simulink model "amalifuzzypidzoptimal"  (R2021a)
settings: Solver=FixedStepAuto  StartTime=0.0  StopTime=60  RelTol=1e-2
InitFcn:
  | Ts=0.01;
  | 
  | Kpmin1 = 3;
  | Kpmax1 = 12;
  | Kdmin1 = 3;
  | Kdmax1 = 11;
  | 
  | Kpmin2 = 3;
  | Kpmax2 = 11;
  | Kdmin2 = 3;
  | Kdmax2 = 10;
  | 
  | Kpmin = 3;
  | Kpmax = 13;
  | Kdmin = 4;
  | Kdmax = 12;
libraries: raspberrypiCommlib x6, pid_lib x4, raspberrypiBasiclib x4, fuzblock x3, simulink_extras x2, etargetslib x1, raspberrypiNetworklib x1
settings Model: Creator=pouria  LastModifiedBy=pouria
settings SolverCC: AlgebraicLoopSolver=TrustRegion  PositivePriorityOrder=on  AutoInsertRateTranBlk=on
settings DataIOCC: LimitDataPoints=on  SaveFormat=Array  ReturnWorkspaceOutputs=off
settings OptimizationCC: EnhancedBackFolding=on  PassReuseOutputArgsAs=Individual arguments  ZeroExternalMemoryAtStartup=off  ZeroInternalMemoryAtStartup=off  MaxStackSize=64  OptimizeBlockOrder=speed  DifferentSizesBufferReuse=on  OptimizationCustomize=off  EfficientTunableParamExpr=on
settings DebuggingCC: ParameterTunabilityLossMsg=error  SFUnexpectedBacktrackingDiag=warning  SFNoUnconditionalDefaultTransitionDiag=warning  SFExecutionAtInitializationDiag=none  SFMachineParentedDataDiag=warning  ArithmeticOperatorsInVariantConditions=warning
settings HardwareCC: ProdBitPerPointer=32  ProdBitPerSizeT=32  ProdBitPerPtrDiffT=32  ProdLargestAtomicInteger=Long  ProdLargestAtomicFloat=Double  ProdWordSize=32  ProdLongLongMode=on  ProdHWDeviceType=ARM Compatible->ARM Cortex
settings ModelReferenceCC: PropagateSignalLabelsOutOfModel=off
settings SFSimCC: SimUseLocalCustomCode=off  CustomCodeUndefinedFunction=UseInterfaceOnly
settings RTWCC: SystemTargetFile=ert.tlc  HardwareBoard=Raspberry Pi  TLCOptions="-aInlineSetEventsForThisBaseRateFcn=TLC_FALSE -aSuppressMultiTaskScheduler=TLC_FALSE  -aRateBasedStepFcn=0"  TemplateMakefile=ert_default_tmf  RTWUseLocalCustomCode=off  Toolchain=GNU GCC Embedded Linux  BuildConfiguration=Faster Runs
settings CodeAppCC: ForceParamTrailComments=on  IgnoreCustomStorageClasses=off  OperatorAnnotations=on  SimulinkDataObjDesc=on  SFDataObjDesc=on  InsertBlockDesc=on
settings ERTTargetCC: SupportContinuousTime=on  SupportVariableSizeSignals=on  ExtModeTransport=2  ExtModeStaticAlloc=on  ExtModeMexFile=ext_xcp  ExtModeIntrfLevel=Level2 - Open
settings ConfigComp: CovMetricSettings=dw  CovSaveCumulativeToWorkspaceVar=on  CovSaveSingleToWorkspaceVar=on  CovExternalEMLEnable=off  CovSFcnEnable=off

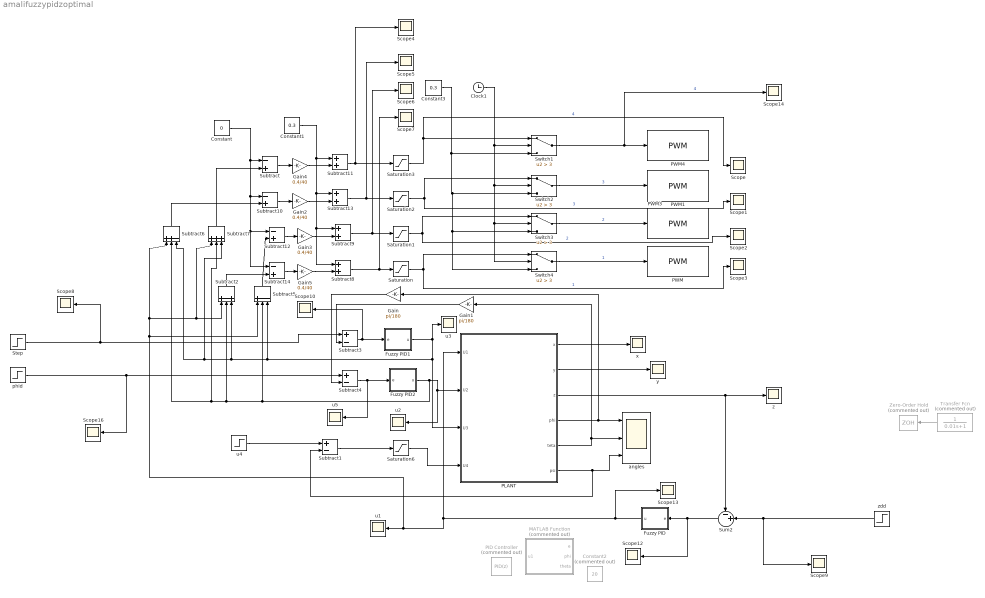
== system amalifuzzypidzoptimal ==
  Clock1 : Clock
  Constant : Constant  Value=0  SampleTime=Ts
  Constant1 : Constant  Value=0.3  SampleTime=Ts
  Constant2 : Constant  Commented=on  Value=20
  Constant3 : Constant  Value=0.3  SampleTime=Ts
  Fuzzy PID : Subsystem
  Fuzzy PID1 : Subsystem
  Fuzzy PID2 : Subsystem
  Gain : Gain  Gain=pi/180
  Gain1 : Gain  Gain=pi/180
  Gain{2..5} (4 alike) : Gain  Gain=0.4/40
  MATLAB Function : MATLAB Function  Commented=on  TreatAsAtomicUnit=on
  PID Controller : pid_lib/PID Controller  Commented=on  Controller=PID  Form=Parallel  TimeDomain=Discrete-time  UseExternalTs=off  SampleTime=0.01  IntegratorMethod=Backward Euler  FilterMethod=Backward Euler  ControllerParametersSource=internal  P=5  I=3  D=5  UseFilter=on  N=100  TunerSelectOption=Transfer Function Based (PID Tuner App)  InitialConditionSource=internal  InitialConditionForIntegrator=0  InitialConditionForFilter=0  DifferentiatorICPrevScaledInput=0  ExternalReset=none  TrackingMode=off  Kt=1  LimitOutput=off  SatLimitsSource=internal  UpperSaturationLimit=inf  LowerSaturationLimit=-inf  LinearizeAsGain=on  AntiWindupMode=none  Kb=1  POutMin=[]  POutMax=[]  IOutMin=[]  IOutMax=[]  DOutMin=[]  DOutMax=[]  NOutMin=[]  NOutMax=[]  SumOutMin=[]  SumOutMax=[]  SaturationOutMin=[]  SaturationOutMax=[]  PParamMin=[]  PParamMax=[]  IParamMin=[]  IParamMax=[]  DParamMin=[]  DParamMax=[]  NParamMin=[]  NParamMax=[]  KbParamMin=[]  KbParamMax=[]  KtParamMin=[]  KtParamMax=[]  KbOutMin=[]  KbOutMax=[]  KtOutMin=[]  KtOutMax=[]  IntegratorOutMin=[]  IntegratorOutMax=[]  FilterOutMin=[]  FilterOutMax=[]  SumI1OutMin=[]  SumI1OutMax=[]  SumI2OutMin=[]  SumI2OutMax=[]  SumI3OutMin=[]  SumI3OutMax=[]  SumI4OutMin=[]  SumI4OutMax=[]  SumDOutMin=[]  SumDOutMax=[]  DifferentiatorOutMin=[]  DifferentiatorOutMax=[]  FilterDiffOutCoefMin=[]  FilterDiffOutCoefMax=[]  ReciprocalOutMin=[]  ReciprocalOutMax=[]  SumDenOutMin=[]  SumDenOutMax=[]  SumNumOutMin=[]  SumNumOutMax=[]  DivideOutMin=[]  DivideOutMax=[]  UdiffTsProdOutMin=[]  UdiffTsProdOutMax=[]  NTsProdOutMin=[]  NTsProdOutMax=[]  UintegralTsProdOutMin=[]  UintegralTsProdOutMax=[]  UngainTsProdOutMin=[]  UngainTsProdOutMax=[]  IntegratorContinuousStateAttributes=''  IntegratorStateMustResolveToSignalObject=off  IntegratorRTWStateStorageClass=Auto  FilterContinuousStateAttributes=''  FilterStateMustResolveToSignalObject=off  FilterRTWStateStorageClass=Auto  ParallelPVariant=InternalParameters  IdealPVariant=Disabled  IVariant=InternalParameters  DVariant=InternalParameters  IntegratorVariant=Discrete  SatVariant=Disabled  AWVariant=Passthrough  PCopyVariant=Disabled  TRVariant=Disabled  FdbkBlocksVariant=Forward  IdealPFdbkVariant=Disabled  SatFdbkVariant=Disabled  DerivativeFilterVariant=BackwardEulerFilter  NVariant=InternalParameters  NCopyVariant=InternalParameters  FilterICVariant=InternalICsFilter  IntegratorICVariant=InternalICs  ExternalResetVariant=Disabled  TRSumVariant=Passthrough  SumFdbkVariant=Disabled  SumVariant=Sum_PID  TsampFilterVariant=InternalTs  TsampNgainVariant=Passthrough  TsampIntegralVariant=Passthrough  ExternalSaturationOutDataTypeStr=Inherit: Same as second input
  PLANT : Subsystem
  PWM : raspberrypiBasiclib/PWM  board=Pi 3 Model B  Pin_=21  Frequency=400  blockPlatform=Raspberry Pi
      settings: SourceProductBaseCode=RASPPI
  PWM1 : raspberrypiBasiclib/PWM  board=Pi 3 Model B  Pin_=20  Frequency=400  blockPlatform=Raspberry Pi
      settings: SourceProductBaseCode=RASPPI
  PWM3 : raspberrypiBasiclib/PWM  board=Pi 3 Model B  Pin_=16  Frequency=400  blockPlatform=Raspberry Pi
      settings: SourceProductBaseCode=RASPPI
  PWM4 : raspberrypiBasiclib/PWM  board=Pi 3 Model B  Pin_=19  Frequency=400  blockPlatform=Raspberry Pi
      settings: SourceProductBaseCode=RASPPI
  Saturation{,1..3} (4 alike) : Saturate  UpperLimit=0.7  LowerLimit=0.3
  Saturation6 : Saturate  UpperLimit=0  LowerLimit=0
  Scope{,1..10,12..14,16} (15 alike) : Scope
  Step : Step  Time=0  After=0  SampleTime=Ts
  Subtract{,10,12,14} (4 alike) : Sum  Inputs=-+
  Subtract1 : Sum  Inputs=+-
  Subtract{8..9,11,13} (4 alike) : Sum
  Subtract2 : Sum  Inputs=+-+
  Subtract3 : Sum  Inputs=+-
  Subtract4 : Sum  Inputs=+-
  Subtract5 : Sum  Inputs=+--
  Subtract6 : Sum  Inputs=++-
  Subtract7 : Sum  Inputs=+++
  Sum2 : Sum  Inputs=-+|
  Switch{1..4} (4 alike) : Switch  Criteria=u2 > Threshold  Threshold=3
  Transfer Fcn : TransferFcn  Commented=on  Denominator=[0.01 1]
  Zero-Order Hold : ZeroOrderHold  Commented=on  SampleTime=Ts
  angles : Scope  NumInputPorts=3
  phid : Step  Time=0  After=0  SampleTime=Ts
  u{1..3,5} (4 alike) : Scope
  u4 : Step  Time=0  After=0  SampleTime=Ts
  x : Scope
  y : Scope
  z : Scope
  zdd : Step  Time=5  Before=0.06  After=0.25  SampleTime=Ts
  wires:
  PLANT/6(psi) -> angles/3, Subtract1/2
  PLANT/1(x) -> x/1
  PLANT/2(y) -> y/1
  Subtract4/1 -> Fuzzy PID2/1(e), u5/1
  Subtract3/1 -> Fuzzy PID1/1(e), Scope10/1
  u4/1 -> Subtract1/1
  Subtract1/1 -> Saturation6/1
  PLANT/3(z) -> z/1, Sum2/1
  PLANT/4(phi) -> angles/1, Gain/1
  PLANT/5(teta) -> angles/2, Gain1/1
  Saturation/1 -> Switch4/1, Scope3/1  "1"
  Saturation1/1 -> Switch3/1, Scope2/1  "2"
  Saturation2/1 -> Switch2/1, Scope1/1  "3"
  Saturation3/1 -> Switch1/1, Scope/1  "4"
  Gain/1 -> Subtract4/2
  Gain1/1 -> Subtract3/2
  Saturation6/1 -> PLANT/4(U4)
  Subtract7/1 -> Subtract/2
  Subtract6/1 -> Subtract10/2
  Subtract5/1 -> Subtract12/2
  Constant/1 -> Subtract14/1, Subtract12/1, Subtract10/1, Subtract/1
  Subtract2/1 -> Subtract14/2
  Clock1/1 -> Switch4/2, Switch3/2, Switch2/2, Switch1/2
  Switch1/1 -> Scope14/1, PWM4/1  "4"
  Constant3/1 -> Switch1/3, Switch3/3, Switch4/3, Switch2/3
  Switch2/1 -> PWM1/1  "3"
  Switch3/1 -> PWM3/1  "2"
  Switch4/1 -> PWM/1  "1"
  Subtract9/1 -> Scope6/1, Saturation1/1
  Subtract13/1 -> Scope5/1, Saturation2/1
  Subtract11/1 -> Scope4/1, Saturation3/1
  Subtract8/1 -> Scope7/1, Saturation/1
  Subtract14/1 -> Gain5/1
  Subtract12/1 -> Gain3/1
  Subtract10/1 -> Gain2/1
  Subtract/1 -> Gain4/1
  Constant1/1 -> Subtract8/1, Subtract9/1, Subtract13/1, Subtract11/1
  Gain4/1 -> Subtract11/2
  Gain2/1 -> Subtract13/2
  Gain3/1 -> Subtract9/2
  Gain5/1 -> Subtract8/2
  Step/1 -> Scope8/1, Subtract3/1
  phid/1 -> Scope16/1, Subtract4/1
  Sum2/1 -> Fuzzy PID/1(e), Scope12/1
  Fuzzy PID1/1(u) -> PLANT/3(U3), Subtract5/3, Subtract2/3, Subtract6/3, Subtract7/3, u3/1
  Fuzzy PID2/1(u) -> u2/1, PLANT/2(U2), Subtract5/2, Subtract2/2, Subtract7/2, Subtract6/2
  Fuzzy PID/1(u) -> Scope13/1, Subtract5/1, Subtract2/1, Subtract7/1, Subtract6/1, u1/1, PLANT/1(U1)
  zdd/1 -> Scope9/1, Sum2/2
  Transfer Fcn/1 -> Zero-Order Hold/1

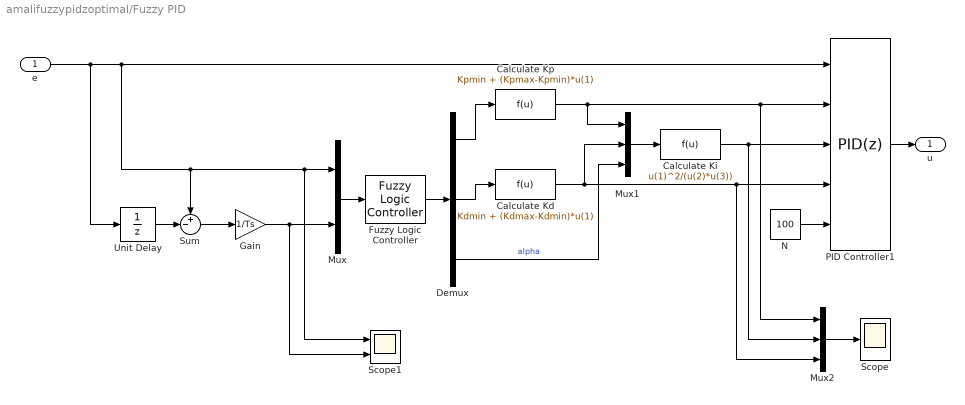
== system amalifuzzypidzoptimal/Fuzzy PID ==
  e : Inport
  Calculate Kd : Fcn  Expr=Kdmin + (Kdmax-Kdmin)*u(1)
  Calculate Ki : Fcn  Expr=u(1)^2/(u(2)*u(3))
  Calculate Kp : Fcn  Expr=Kpmin + (Kpmax-Kpmin)*u(1)
  Demux : Demux  Outputs=3
  Fuzzy Logic Controller : fuzblock/Fuzzy Logic  Controller  FIS='fuzzy_pid1.fis'  OutputSampleNumber=101  DataType=double  FuzzifiedInputs=off  RuleFiringStrengths=off  RuleOutputs=off  AggregatedOutputs=off  SimulateUsing=Interpreted execution  OutOfRangeInputValueMessage=warning  NoRuleFiredMessage=warning  EmptyOutputFuzzySetMessage=warning
  Gain : Gain  Gain=1/Ts
  Mux : Mux  Inputs=2
  Mux1 : Mux  Inputs=3
  Mux2 : Mux  Inputs=3
  N : Constant  Value=100
  PID Controller1 : pid_lib/PID Controller  Controller=PID  Form=Parallel  TimeDomain=Discrete-time  UseExternalTs=off  SampleTime=Ts  IntegratorMethod=Backward Euler  FilterMethod=Backward Euler  ControllerParametersSource=external  P=0.6*4.6737  I=1.2*4.6737/3.26  D=0.6*4.6737*3.26/8  UseFilter=on  N=100  TunerSelectOption=Transfer Function Based (PID Tuner App)  InitialConditionSource=internal  InitialConditionForIntegrator=0  InitialConditionForFilter=0  DifferentiatorICPrevScaledInput=0  ExternalReset=none  TrackingMode=off  Kt=1  LimitOutput=off  SatLimitsSource=internal  UpperSaturationLimit=inf  LowerSaturationLimit=-inf  LinearizeAsGain=on  AntiWindupMode=none  Kb=1  POutMin=[]  POutMax=[]  IOutMin=[]  IOutMax=[]  DOutMin=[]  DOutMax=[]  NOutMin=[]  NOutMax=[]  SumOutMin=[]  SumOutMax=[]  SaturationOutMin=[]  SaturationOutMax=[]  PParamMin=[]  PParamMax=[]  IParamMin=[]  IParamMax=[]  DParamMin=[]  DParamMax=[]  NParamMin=[]  NParamMax=[]  KbParamMin=[]  KbParamMax=[]  KtParamMin=[]  KtParamMax=[]  KbOutMin=[]  KbOutMax=[]  KtOutMin=[]  KtOutMax=[]  IntegratorOutMin=[]  IntegratorOutMax=[]  FilterOutMin=[]  FilterOutMax=[]  SumI1OutMin=[]  SumI1OutMax=[]  SumI2OutMin=[]  SumI2OutMax=[]  SumI3OutMin=[]  SumI3OutMax=[]  SumI4OutMin=[]  SumI4OutMax=[]  SumDOutMin=[]  SumDOutMax=[]  DifferentiatorOutMin=[]  DifferentiatorOutMax=[]  FilterDiffOutCoefMin=[]  FilterDiffOutCoefMax=[]  ReciprocalOutMin=[]  ReciprocalOutMax=[]  SumDenOutMin=[]  SumDenOutMax=[]  SumNumOutMin=[]  SumNumOutMax=[]  DivideOutMin=[]  DivideOutMax=[]  UdiffTsProdOutMin=[]  UdiffTsProdOutMax=[]  NTsProdOutMin=[]  NTsProdOutMax=[]  UintegralTsProdOutMin=[]  UintegralTsProdOutMax=[]  UngainTsProdOutMin=[]  UngainTsProdOutMax=[]  IntegratorContinuousStateAttributes=''  IntegratorStateMustResolveToSignalObject=off  IntegratorRTWStateStorageClass=Auto  FilterContinuousStateAttributes=''  FilterStateMustResolveToSignalObject=off  FilterRTWStateStorageClass=Auto  ParallelPVariant=ExternalParameters  IdealPVariant=Disabled  IVariant=ExternalParameters  DVariant=ExternalParameters  IntegratorVariant=Discrete  SatVariant=Disabled  AWVariant=Passthrough  PCopyVariant=Disabled  TRVariant=Disabled  FdbkBlocksVariant=Forward  IdealPFdbkVariant=Disabled  SatFdbkVariant=Disabled  DerivativeFilterVariant=BackwardEulerFilter  NVariant=ExternalParameters  NCopyVariant=ExternalParameters  FilterICVariant=InternalICsFilter  IntegratorICVariant=InternalICs  ExternalResetVariant=Disabled  TRSumVariant=Passthrough  SumFdbkVariant=Disabled  SumVariant=Sum_PID  TsampFilterVariant=InternalTs  TsampNgainVariant=Passthrough  TsampIntegralVariant=Passthrough  ExternalSaturationOutDataTypeStr=Inherit: Same as second input
  Scope : Scope
  Scope1 : Scope  NumInputPorts=2
  Sum : Sum  Inputs=+-|
  Unit Delay : UnitDelay  SampleTime=Ts  HasFrameUpgradeWarning=on
  u : Outport
  wires:
  PID Controller1/1 -> u/1
  N/1 -> PID Controller1/5
  Mux/1 -> Fuzzy Logic Controller/1
  Fuzzy Logic Controller/1 -> Demux/1
  Demux/1 -> Calculate Kp/1
  Calculate Kp/1 -> Mux2/1, PID Controller1/2, Mux1/1
  Demux/2 -> Calculate Kd/1
  Calculate Kd/1 -> Mux1/2, Mux2/3, PID Controller1/4
  Calculate Ki/1 -> Mux2/2, PID Controller1/3
  Mux1/1 -> Calculate Ki/1
  Demux/3 -> Mux1/3  "alpha"
  Unit Delay/1 -> Sum/2
  Mux2/1 -> Scope/1
  e/1 -> Unit Delay/1, Sum/1, Scope1/1, Mux/1, PID Controller1/1
  Sum/1 -> Gain/1
  Gain/1 -> Scope1/2, Mux/2

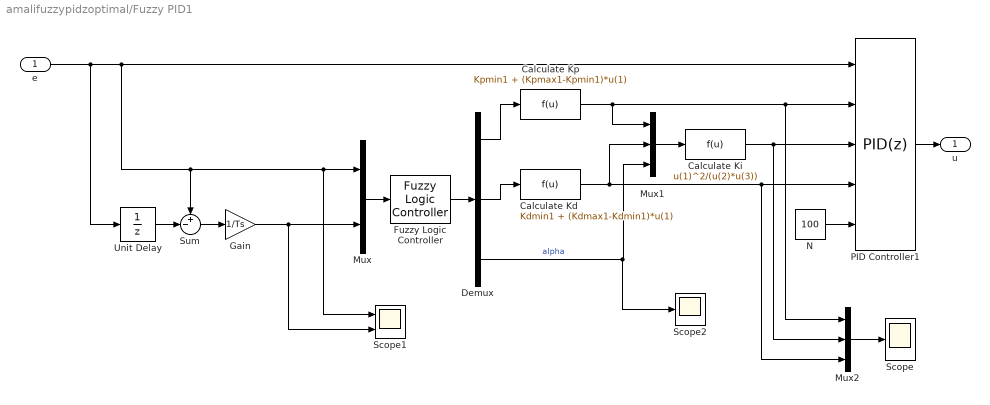
== system amalifuzzypidzoptimal/Fuzzy PID1 ==
  e : Inport
  Calculate Kd : Fcn  Expr=Kdmin1 + (Kdmax1-Kdmin1)*u(1)
  Calculate Ki : Fcn  Expr=u(1)^2/(u(2)*u(3))
  Calculate Kp : Fcn  Expr=Kpmin1 + (Kpmax1-Kpmin1)*u(1)
  Demux : Demux  Outputs=3
  Fuzzy Logic Controller : fuzblock/Fuzzy Logic  Controller  FIS='fuzzy_pidzavie.fis'  OutputSampleNumber=101  DataType=double  FuzzifiedInputs=off  RuleFiringStrengths=off  RuleOutputs=off  AggregatedOutputs=off  SimulateUsing=Interpreted execution  OutOfRangeInputValueMessage=warning  NoRuleFiredMessage=warning  EmptyOutputFuzzySetMessage=warning
  Gain : Gain  Gain=1/Ts
  Mux : Mux  Inputs=2
  Mux1 : Mux  Inputs=3
  Mux2 : Mux  Inputs=3
  N : Constant  Value=100
  PID Controller1 : pid_lib/PID Controller  Controller=PID  Form=Parallel  TimeDomain=Discrete-time  UseExternalTs=off  SampleTime=Ts  IntegratorMethod=Backward Euler  FilterMethod=Backward Euler  ControllerParametersSource=external  P=0.6*4.6737  I=1.2*4.6737/3.26  D=0.6*4.6737*3.26/8  UseFilter=on  N=100  TunerSelectOption=Transfer Function Based (PID Tuner App)  InitialConditionSource=internal  InitialConditionForIntegrator=0  InitialConditionForFilter=0  DifferentiatorICPrevScaledInput=0  ExternalReset=none  TrackingMode=off  Kt=1  LimitOutput=off  SatLimitsSource=internal  UpperSaturationLimit=inf  LowerSaturationLimit=-inf  LinearizeAsGain=on  AntiWindupMode=none  Kb=1  POutMin=[]  POutMax=[]  IOutMin=[]  IOutMax=[]  DOutMin=[]  DOutMax=[]  NOutMin=[]  NOutMax=[]  SumOutMin=[]  SumOutMax=[]  SaturationOutMin=[]  SaturationOutMax=[]  PParamMin=[]  PParamMax=[]  IParamMin=[]  IParamMax=[]  DParamMin=[]  DParamMax=[]  NParamMin=[]  NParamMax=[]  KbParamMin=[]  KbParamMax=[]  KtParamMin=[]  KtParamMax=[]  KbOutMin=[]  KbOutMax=[]  KtOutMin=[]  KtOutMax=[]  IntegratorOutMin=[]  IntegratorOutMax=[]  FilterOutMin=[]  FilterOutMax=[]  SumI1OutMin=[]  SumI1OutMax=[]  SumI2OutMin=[]  SumI2OutMax=[]  SumI3OutMin=[]  SumI3OutMax=[]  SumI4OutMin=[]  SumI4OutMax=[]  SumDOutMin=[]  SumDOutMax=[]  DifferentiatorOutMin=[]  DifferentiatorOutMax=[]  FilterDiffOutCoefMin=[]  FilterDiffOutCoefMax=[]  ReciprocalOutMin=[]  ReciprocalOutMax=[]  SumDenOutMin=[]  SumDenOutMax=[]  SumNumOutMin=[]  SumNumOutMax=[]  DivideOutMin=[]  DivideOutMax=[]  UdiffTsProdOutMin=[]  UdiffTsProdOutMax=[]  NTsProdOutMin=[]  NTsProdOutMax=[]  UintegralTsProdOutMin=[]  UintegralTsProdOutMax=[]  UngainTsProdOutMin=[]  UngainTsProdOutMax=[]  IntegratorContinuousStateAttributes=''  IntegratorStateMustResolveToSignalObject=off  IntegratorRTWStateStorageClass=Auto  FilterContinuousStateAttributes=''  FilterStateMustResolveToSignalObject=off  FilterRTWStateStorageClass=Auto  ParallelPVariant=ExternalParameters  IdealPVariant=Disabled  IVariant=ExternalParameters  DVariant=ExternalParameters  IntegratorVariant=Discrete  SatVariant=Disabled  AWVariant=Passthrough  PCopyVariant=Disabled  TRVariant=Disabled  FdbkBlocksVariant=Forward  IdealPFdbkVariant=Disabled  SatFdbkVariant=Disabled  DerivativeFilterVariant=BackwardEulerFilter  NVariant=ExternalParameters  NCopyVariant=ExternalParameters  FilterICVariant=InternalICsFilter  IntegratorICVariant=InternalICs  ExternalResetVariant=Disabled  TRSumVariant=Passthrough  SumFdbkVariant=Disabled  SumVariant=Sum_PID  TsampFilterVariant=InternalTs  TsampNgainVariant=Passthrough  TsampIntegralVariant=Passthrough  ExternalSaturationOutDataTypeStr=Inherit: Same as second input
  Scope : Scope
  Scope1 : Scope  NumInputPorts=2
  Scope2 : Scope
  Sum : Sum  Inputs=+-|
  Unit Delay : UnitDelay  SampleTime=Ts  HasFrameUpgradeWarning=on
  u : Outport
  wires:
  PID Controller1/1 -> u/1
  N/1 -> PID Controller1/5
  Mux/1 -> Fuzzy Logic Controller/1
  Fuzzy Logic Controller/1 -> Demux/1
  Demux/1 -> Calculate Kp/1
  Calculate Kp/1 -> Mux2/1, PID Controller1/2, Mux1/1
  Demux/2 -> Calculate Kd/1
  Calculate Kd/1 -> Mux1/2, Mux2/3, PID Controller1/4
  Calculate Ki/1 -> Mux2/2, PID Controller1/3
  Mux1/1 -> Calculate Ki/1
  Demux/3 -> Scope2/1, Mux1/3  "alpha"
  Unit Delay/1 -> Sum/2
  Mux2/1 -> Scope/1
  e/1 -> Unit Delay/1, Sum/1, Scope1/1, Mux/1, PID Controller1/1
  Sum/1 -> Gain/1
  Gain/1 -> Scope1/2, Mux/2

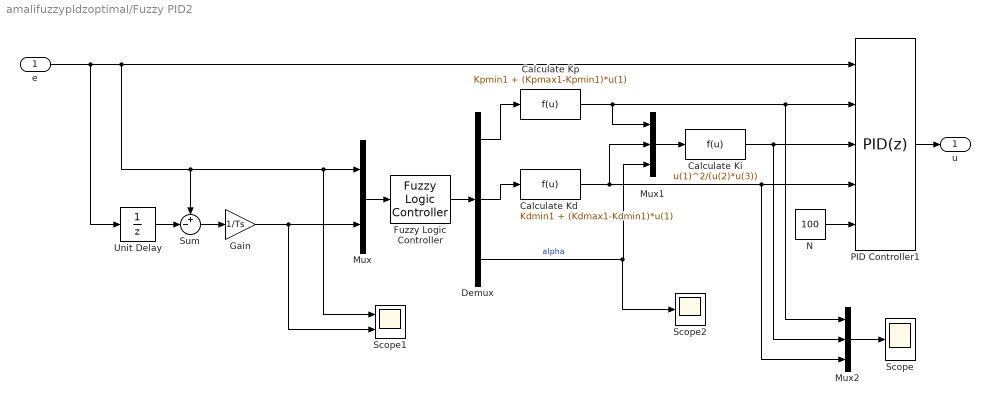
== system amalifuzzypidzoptimal/Fuzzy PID2 ==
  e : Inport
  Calculate Kd : Fcn  Expr=Kdmin1 + (Kdmax1-Kdmin1)*u(1)
  Calculate Ki : Fcn  Expr=u(1)^2/(u(2)*u(3))
  Calculate Kp : Fcn  Expr=Kpmin1 + (Kpmax1-Kpmin1)*u(1)
  Demux : Demux  Outputs=3
  Fuzzy Logic Controller : fuzblock/Fuzzy Logic  Controller  FIS='fuzzy_pidzavie.fis'  OutputSampleNumber=101  DataType=double  FuzzifiedInputs=off  RuleFiringStrengths=off  RuleOutputs=off  AggregatedOutputs=off  SimulateUsing=Interpreted execution  OutOfRangeInputValueMessage=warning  NoRuleFiredMessage=warning  EmptyOutputFuzzySetMessage=warning
  Gain : Gain  Gain=1/Ts
  Mux : Mux  Inputs=2
  Mux1 : Mux  Inputs=3
  Mux2 : Mux  Inputs=3
  N : Constant  Value=100
  PID Controller1 : pid_lib/PID Controller  Controller=PID  Form=Parallel  TimeDomain=Discrete-time  UseExternalTs=off  SampleTime=Ts  IntegratorMethod=Backward Euler  FilterMethod=Backward Euler  ControllerParametersSource=external  P=0.6*4.6737  I=1.2*4.6737/3.26  D=0.6*4.6737*3.26/8  UseFilter=on  N=100  TunerSelectOption=Transfer Function Based (PID Tuner App)  InitialConditionSource=internal  InitialConditionForIntegrator=0  InitialConditionForFilter=0  DifferentiatorICPrevScaledInput=0  ExternalReset=none  TrackingMode=off  Kt=1  LimitOutput=off  SatLimitsSource=internal  UpperSaturationLimit=inf  LowerSaturationLimit=-inf  LinearizeAsGain=on  AntiWindupMode=none  Kb=1  POutMin=[]  POutMax=[]  IOutMin=[]  IOutMax=[]  DOutMin=[]  DOutMax=[]  NOutMin=[]  NOutMax=[]  SumOutMin=[]  SumOutMax=[]  SaturationOutMin=[]  SaturationOutMax=[]  PParamMin=[]  PParamMax=[]  IParamMin=[]  IParamMax=[]  DParamMin=[]  DParamMax=[]  NParamMin=[]  NParamMax=[]  KbParamMin=[]  KbParamMax=[]  KtParamMin=[]  KtParamMax=[]  KbOutMin=[]  KbOutMax=[]  KtOutMin=[]  KtOutMax=[]  IntegratorOutMin=[]  IntegratorOutMax=[]  FilterOutMin=[]  FilterOutMax=[]  SumI1OutMin=[]  SumI1OutMax=[]  SumI2OutMin=[]  SumI2OutMax=[]  SumI3OutMin=[]  SumI3OutMax=[]  SumI4OutMin=[]  SumI4OutMax=[]  SumDOutMin=[]  SumDOutMax=[]  DifferentiatorOutMin=[]  DifferentiatorOutMax=[]  FilterDiffOutCoefMin=[]  FilterDiffOutCoefMax=[]  ReciprocalOutMin=[]  ReciprocalOutMax=[]  SumDenOutMin=[]  SumDenOutMax=[]  SumNumOutMin=[]  SumNumOutMax=[]  DivideOutMin=[]  DivideOutMax=[]  UdiffTsProdOutMin=[]  UdiffTsProdOutMax=[]  NTsProdOutMin=[]  NTsProdOutMax=[]  UintegralTsProdOutMin=[]  UintegralTsProdOutMax=[]  UngainTsProdOutMin=[]  UngainTsProdOutMax=[]  IntegratorContinuousStateAttributes=''  IntegratorStateMustResolveToSignalObject=off  IntegratorRTWStateStorageClass=Auto  FilterContinuousStateAttributes=''  FilterStateMustResolveToSignalObject=off  FilterRTWStateStorageClass=Auto  ParallelPVariant=ExternalParameters  IdealPVariant=Disabled  IVariant=ExternalParameters  DVariant=ExternalParameters  IntegratorVariant=Discrete  SatVariant=Disabled  AWVariant=Passthrough  PCopyVariant=Disabled  TRVariant=Disabled  FdbkBlocksVariant=Forward  IdealPFdbkVariant=Disabled  SatFdbkVariant=Disabled  DerivativeFilterVariant=BackwardEulerFilter  NVariant=ExternalParameters  NCopyVariant=ExternalParameters  FilterICVariant=InternalICsFilter  IntegratorICVariant=InternalICs  ExternalResetVariant=Disabled  TRSumVariant=Passthrough  SumFdbkVariant=Disabled  SumVariant=Sum_PID  TsampFilterVariant=InternalTs  TsampNgainVariant=Passthrough  TsampIntegralVariant=Passthrough  ExternalSaturationOutDataTypeStr=Inherit: Same as second input
  Scope : Scope
  Scope1 : Scope  NumInputPorts=2
  Scope2 : Scope
  Sum : Sum  Inputs=+-|
  Unit Delay : UnitDelay  SampleTime=Ts  HasFrameUpgradeWarning=on
  u : Outport
  wires:
  PID Controller1/1 -> u/1
  N/1 -> PID Controller1/5
  Mux/1 -> Fuzzy Logic Controller/1
  Fuzzy Logic Controller/1 -> Demux/1
  Demux/1 -> Calculate Kp/1
  Calculate Kp/1 -> Mux2/1, PID Controller1/2, Mux1/1
  Demux/2 -> Calculate Kd/1
  Calculate Kd/1 -> Mux1/2, Mux2/3, PID Controller1/4
  Calculate Ki/1 -> Mux2/2, PID Controller1/3
  Mux1/1 -> Calculate Ki/1
  Demux/3 -> Scope2/1, Mux1/3  "alpha"
  Unit Delay/1 -> Sum/2
  Mux2/1 -> Scope/1
  e/1 -> Unit Delay/1, Sum/1, Scope1/1, Mux/1, PID Controller1/1
  Sum/1 -> Gain/1
  Gain/1 -> Scope1/2, Mux/2

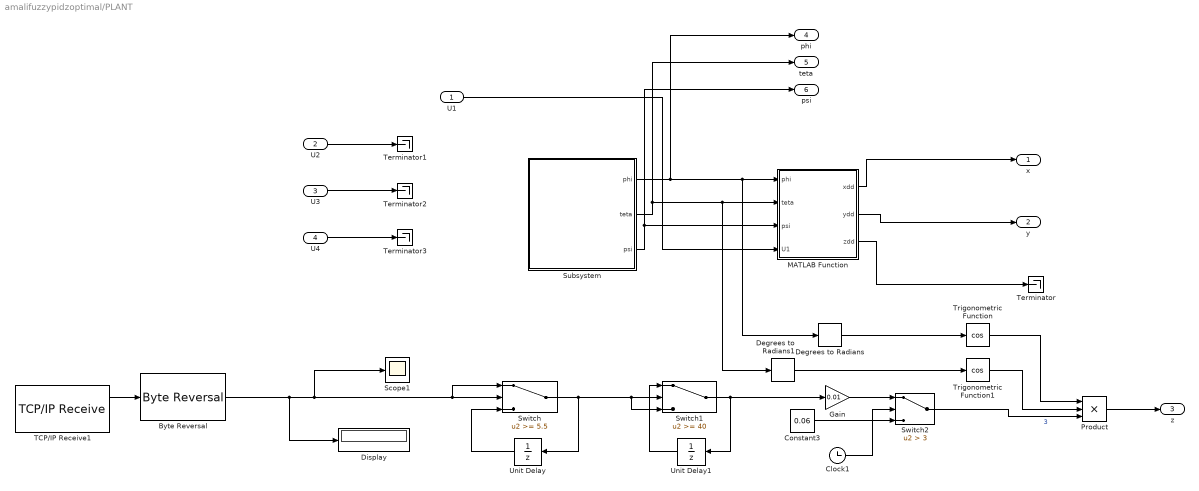
== system amalifuzzypidzoptimal/PLANT ==
  U1 : Inport
  U2 : Inport  Port=2
  U3 : Inport  Port=3
  U4 : Inport  Port=4
  Byte Reversal : etargetslib/Byte Reversal  numInp=1
      settings: SourceProductBaseCode=ME
  Clock1 : Clock
  Constant3 : Constant  Value=0.06  SampleTime=Ts
  Degrees to Radians : simulink_extras/Transformations/Degrees to Radians
  Degrees to Radians1 : simulink_extras/Transformations/Degrees to Radians
  Display : Display
  Gain : Gain  Gain=0.01
  MATLAB Function : MATLAB Function  TreatAsAtomicUnit=on
  Product : Product  Inputs=3
  Scope1 : Scope
  Subsystem : Subsystem
  Switch : Switch  Threshold=5.5
  Switch1 : Switch  Threshold=40
  Switch2 : Switch  Criteria=u2 > Threshold  Threshold=3
  TCP/IP Receive1 : raspberrypiNetworklib/TCP//IP Receive  Mode_=Client  LocalServerPort_=25000  RemoteAddr_=192.168.43.77  RemoteServerPort_=12345  DataType_=double  DataSize_=1  SampleTime_=Ts  SimulateUsing=Code generation  ClientPortBindingSelection_=off  ClientPortToBind_=35000  BlockingMode_=off  BlockTimeout_=0.1  BlockPlatform=RASPBERRYPI
      settings: SourceProductBaseCode=RASPPI
  Terminator{,1..3} (4 alike) : Terminator
  Trigonometric Function : Trigonometry  Operator=cos
  Trigonometric Function1 : Trigonometry  Operator=cos
  Unit Delay : UnitDelay  SampleTime=Ts  HasFrameUpgradeWarning=on
  Unit Delay1 : UnitDelay  SampleTime=Ts  HasFrameUpgradeWarning=on
  x : Outport
  y : Outport  Port=2
  z : Outport  Port=3
  phi : Outport  Port=4
  teta : Outport  Port=5
  psi : Outport  Port=6
  wires:
  MATLAB Function/1(xdd) -> x/1
  U1/1 -> MATLAB Function/4(U1)
  MATLAB Function/2(ydd) -> y/1
  Subsystem/1(phi) -> phi/1, Degrees to Radians/1, MATLAB Function/1(phi)
  Subsystem/2(teta) -> teta/1, Degrees to Radians1/1, MATLAB Function/2(teta)
  Subsystem/3(psi) -> psi/1, MATLAB Function/3(psi)
  MATLAB Function/3(zdd) -> Terminator/1
  TCP/IP Receive1/1 -> Byte Reversal/1
  Clock1/1 -> Switch2/2
  Gain/1 -> Switch2/1
  Constant3/1 -> Switch2/3
  Unit Delay1/1 -> Switch1/1
  Byte Reversal/1 -> Switch/1, Switch/2, Scope1/1, Display/1
  Switch1/1 -> Gain/1, Unit Delay1/1
  Switch/1 -> Unit Delay/1, Switch1/3, Switch1/2
  Unit Delay/1 -> Switch/3
  Degrees to Radians/1 -> Trigonometric Function/1
  Degrees to Radians1/1 -> Trigonometric Function1/1
  Switch2/1 -> Product/3  "3"
  Trigonometric Function1/1 -> Product/2
  Trigonometric Function/1 -> Product/1
  Product/1 -> z/1
  U2/1 -> Terminator1/1
  U3/1 -> Terminator2/1
  U4/1 -> Terminator3/1

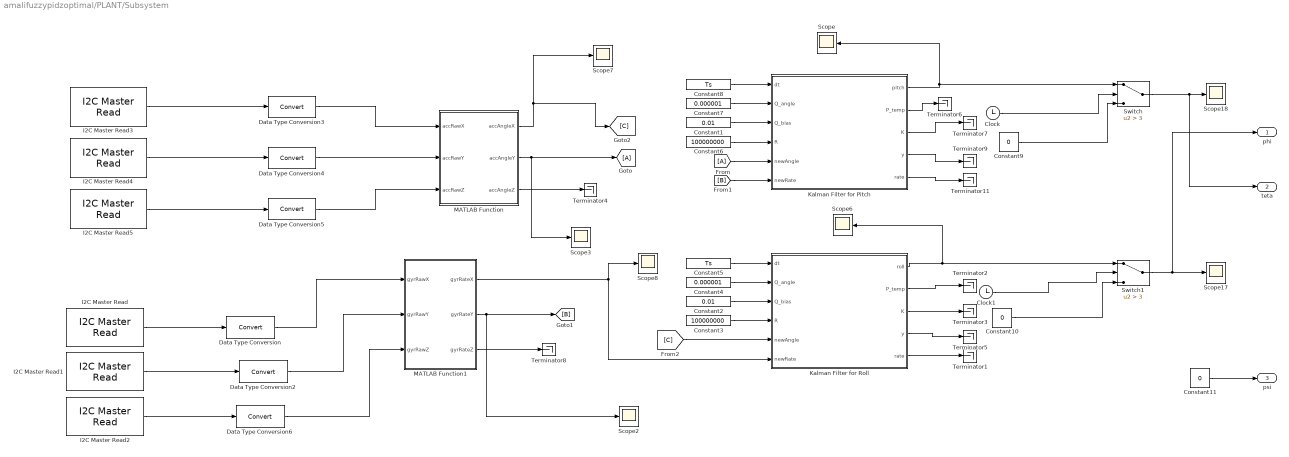
== system amalifuzzypidzoptimal/PLANT/Subsystem ==
  Clock : Clock
  Clock1 : Clock
  Constant1 : Constant  Value=0.01  SampleTime=0.01
  Constant10 : Constant  Value=0  SampleTime=Ts
  Constant11 : Constant  Value=0  SampleTime=Ts
  Constant2 : Constant  Value=0.01  SampleTime=0.01
  Constant3 : Constant  Value=100000000  SampleTime=0.01
  Constant4 : Constant  Value=0.000001  SampleTime=0.01
  Constant5 : Constant  Value=Ts  SampleTime=Ts
  Constant6 : Constant  Value=100000000  SampleTime=0.01
  Constant7 : Constant  Value=0.000001  SampleTime=0.01
  Constant8 : Constant  Value=Ts  SampleTime=Ts
  Constant9 : Constant  Value=0  SampleTime=Ts
  Data Type Conversion{,2..6} (6 alike) : DataTypeConversion
  I2C Master Read : raspberrypiCommlib/I2C Master Read  BoardProperty=Pi 3 Model B+  Mode=Master  SlaveAddress="hex2dec(\"0x68\")"  SlaveByteOrder=BigEndian  Direction=Receiver  RegisterAddressMode=on  RegisterAddress=67  SlaveDataType=int16  DataLength=1  NoAck=off  RepeatedStart=off  OutputStatus=off  SampleTime=Ts
      settings: SourceProductBaseCode=RASPPI
  I2C Master Read1 : raspberrypiCommlib/I2C Master Read  BoardProperty=Pi 3 Model B+  Mode=Master  SlaveAddress="hex2dec(\"0x68\")"  SlaveByteOrder=BigEndian  Direction=Receiver  RegisterAddressMode=on  RegisterAddress=69  SlaveDataType=int16  DataLength=1  NoAck=off  RepeatedStart=off  OutputStatus=off  SampleTime=Ts
      settings: SourceProductBaseCode=RASPPI
  I2C Master Read2 : raspberrypiCommlib/I2C Master Read  BoardProperty=Pi 3 Model B+  Mode=Master  SlaveAddress="hex2dec(\"0x68\")"  SlaveByteOrder=BigEndian  Direction=Receiver  RegisterAddressMode=on  RegisterAddress=71  SlaveDataType=int16  DataLength=1  NoAck=off  RepeatedStart=off  OutputStatus=off  SampleTime=Ts
      settings: SourceProductBaseCode=RASPPI
  I2C Master Read3 : raspberrypiCommlib/I2C Master Read  BoardProperty=Pi 3 Model B+  Mode=Master  SlaveAddress="hex2dec(\"0x68\")"  SlaveByteOrder=BigEndian  Direction=Receiver  RegisterAddressMode=on  RegisterAddress=59  SlaveDataType=int16  DataLength=1  NoAck=off  RepeatedStart=off  OutputStatus=off  SampleTime=Ts
      settings: SourceProductBaseCode=RASPPI
  I2C Master Read4 : raspberrypiCommlib/I2C Master Read  BoardProperty=Pi 3 Model B+  Mode=Master  SlaveAddress="hex2dec(\"0x68\")"  SlaveByteOrder=BigEndian  Direction=Receiver  RegisterAddressMode=on  RegisterAddress=61  SlaveDataType=int16  DataLength=1  NoAck=off  RepeatedStart=off  OutputStatus=off  SampleTime=Ts
      settings: SourceProductBaseCode=RASPPI
  I2C Master Read5 : raspberrypiCommlib/I2C Master Read  BoardProperty=Pi 3 Model B+  Mode=Master  SlaveAddress="hex2dec(\"0x68\")"  SlaveByteOrder=BigEndian  Direction=Receiver  RegisterAddressMode=on  RegisterAddress=63  SlaveDataType=int16  DataLength=1  NoAck=off  RepeatedStart=off  OutputStatus=off  SampleTime=Ts
      settings: SourceProductBaseCode=RASPPI
  Kalman Filter for Pitch : MATLAB Function  TreatAsAtomicUnit=on
  Kalman Filter for Roll : MATLAB Function  TreatAsAtomicUnit=on
  MATLAB Function : MATLAB Function  TreatAsAtomicUnit=on
  MATLAB Function1 : MATLAB Function  TreatAsAtomicUnit=on
  Scope{,2..3,6..8,17..18} (8 alike) : Scope
  Switch : Switch  Criteria=u2 > Threshold  Threshold=3
  Switch1 : Switch  Criteria=u2 > Threshold  Threshold=3
  Terminator{1..9,11} (10 alike) : Terminator
  phi : Outport
  teta : Outport  Port=2
  psi : Outport  Port=3
  wires:
  Clock/1 -> Switch/2
  I2C Master Read1/1 -> Data Type Conversion2/1
  Switch/1 -> teta/1, Scope18/1
  Constant3/1 -> Kalman Filter for Roll/4(R)
  MATLAB Function/2(accAngleY) -> [A], Scope3/1
  Data Type Conversion6/1 -> MATLAB Function1/3(gyrRawZ)
  Switch1/1 -> phi/1, Scope17/1
  MATLAB Function/1(accAngleX) -> [C], Scope7/1
  Kalman Filter for Pitch/1(pitch) -> Switch/1, Scope/1
  Constant9/1 -> Switch/3
  Kalman Filter for Roll/1(roll) -> Switch1/1, Scope6/1
  Kalman Filter for Roll/3(K) -> Terminator3/1
  Clock1/1 -> Switch1/2
  I2C Master Read/1 -> Data Type Conversion/1
  Constant10/1 -> Switch1/3
  Data Type Conversion3/1 -> MATLAB Function/1(accRawX)
  Constant5/1 -> Kalman Filter for Roll/1(dt)
  I2C Master Read2/1 -> Data Type Conversion6/1
  MATLAB Function1/1(gyrRateX) -> Kalman Filter for Roll/6(newRate), Scope8/1
  Kalman Filter for Pitch/4(y) -> Terminator9/1
  Kalman Filter for Pitch/3(K) -> Terminator7/1
  Kalman Filter for Pitch/2(P_temp) -> Terminator6/1
  [A] -> Kalman Filter for Pitch/5(newAngle)
  I2C Master Read3/1 -> Data Type Conversion3/1
  Kalman Filter for Roll/2(P_temp) -> Terminator2/1
  [B] -> Kalman Filter for Pitch/6(newRate)
  Constant7/1 -> Kalman Filter for Pitch/2(Q_angle)
  [C] -> Kalman Filter for Roll/5(newAngle)
  Data Type Conversion/1 -> MATLAB Function1/1(gyrRawX)
  Data Type Conversion2/1 -> MATLAB Function1/2(gyrRawY)
  Kalman Filter for Roll/5(rate) -> Terminator1/1
  Constant6/1 -> Kalman Filter for Pitch/4(R)
  Constant8/1 -> Kalman Filter for Pitch/1(dt)
  Constant2/1 -> Kalman Filter for Roll/3(Q_bias)
  Constant4/1 -> Kalman Filter for Roll/2(Q_angle)
  I2C Master Read5/1 -> Data Type Conversion5/1
  Kalman Filter for Pitch/5(rate) -> Terminator11/1
  Data Type Conversion5/1 -> MATLAB Function/3(accRawZ)
  MATLAB Function1/2(gyrRateY) -> [B], Scope2/1
  Data Type Conversion4/1 -> MATLAB Function/2(accRawY)
  I2C Master Read4/1 -> Data Type Conversion4/1
  Kalman Filter for Roll/4(y) -> Terminator5/1
  Constant1/1 -> Kalman Filter for Pitch/3(Q_bias)
  Constant11/1 -> psi/1
  MATLAB Function/3(accAngleZ) -> Terminator4/1
  MATLAB Function1/3(gyrRateZ) -> Terminator8/1

== matlab function amalifuzzypidzoptimal/MATLAB Function ==
  data: u1 output; e input; phi input; theta input
function u1 = fcn(e,phi,theta)
%#codegen
m=1.1;
u1=(e+9.81)*m/(abs(cosd(phi)*cosd(theta)));

== matlab function amalifuzzypidzoptimal/PLANT/Subsystem/MATLAB Function ==
  data: accRawX input; accAngleX output; accAngleY output; accRawY input; accRawZ input; accAngleZ output
function [accAngleX, accAngleY, accAngleZ] = fcn(accRawX, accRawY, accRawZ)

%Converting the raw accel data from g values to accel about X and Y axis

accAngleX = atan(accRawY/sqrt(power(accRawX,2) + power(accRawZ,2)))*(180/pi);
accAngleY = atan(-1*(accRawX/sqrt(power(accRawY,2) + power(accRawZ,2))))*(180/pi);
accAngleZ = atan(accRawZ/sqrt(power(accRawX,2) + power(accRawZ,2)))*(180/pi);

end

== matlab function amalifuzzypidzoptimal/PLANT/MATLAB Function ==
  data: phi input; xdd output; teta input; psi input; ydd output; zdd output; U1 input
function [xdd,ydd,zdd] = fcn(phi,teta,psi,U1)
%#codegen
m=1.5;
xdd=((cos(phi)*sin(teta)*cos(psi))+(sin(phi)*sin(psi)))*U1/m;
ydd=((cos(phi)*sin(teta)*sin(psi))+(sin(phi)*cos(psi)))*U1/m;
zdd=-9.81+(cos(phi)*cos(teta)*U1/m);
end

== matlab function amalifuzzypidzoptimal/PLANT/Subsystem/MATLAB Function1 ==
  data: gyrRawX input; gyrRateX output; gyrRateY output; gyrRawY input; gyrRawZ input; gyrRateZ output
function [gyrRateX, gyrRateY, gyrRateZ] = fcn(gyrRawX, gyrRawY, gyrRawZ)

gyrRateX = gyrRawX/131.0;
gyrRateY = gyrRawY/131.0;
gyrRateZ = gyrRawZ/131.0;

end

== matlab function amalifuzzypidzoptimal/PLANT/Subsystem/Kalman Filter for Pitch ==
  data: dt input; pitch output; Q_angle input; Q_bias input; R input; newAngle input; newRate input; P_temp output; K output; y output; rate output
function [pitch, P_temp, K, y, rate]  = kalFilterPitch(dt, Q_angle, Q_bias, R, newAngle, newRate)

persistent angle;
persistent P;
persistent bias_p;

%Process Noise Convariance Matrix
Q = [Q_angle 0; 0 Q_bias] * dt;
F = [1  dt; 0 1];
H = [1 0];
% bias = 6.7483;

if isempty(bias_p)
    bias_p = 6.7850;
end

rate = newRate - bias_p;

if isempty(angle); angle = 0;
    
else
    angle = angle + (dt * rate);
end 

pitch = angle;

if isempty(P); P = [0, 0; 0, 0];
else
    P = F*P*F' + Q;
end 
P_temp = P;

S = H*P*H' + R;
K = (P_temp * H')/S;
y = newAngle - pitch; 
pitch = pitch + K(1) * y;
bias_p = bias_p + K(2) * y;
angle = pitch;

I = [1 0; 0 1];
P_temp = (I - K*H)*P_temp;
P = P_temp;

return 


end

== matlab function amalifuzzypidzoptimal/PLANT/Subsystem/Kalman Filter for Roll ==
  data: dt input; roll output; Q_angle input; Q_bias input; R input; newAngle input; newRate input; P_temp output; K output; y output; rate output
function [roll, P_temp, K, y, rate]  = kalFilterRoll(dt, Q_angle, Q_bias, R, newAngle, newRate)

persistent angle;
persistent P;
persistent bias_r;

%Process Noise Convariance Matrix
Q = [Q_angle 0; 0 Q_bias] * dt;
F = [1  dt; 0 1];
H = [1 0];
% bias = 3.3726;

if isempty(bias_r)
    bias_r = 3.7357;
end

rate = newRate - bias_r;

if isempty(angle); angle = 0;
    
else
    angle = angle + (dt * rate);
end 

roll = angle;

if isempty(P); P = [0, 0; 0, 0];
else
    P = F*P*F' + Q;
end 
P_temp = P;

S = H*P*H' + R;
K = (P_temp * H')/S;
y = newAngle - roll; 
roll = roll + K(1) * y;
bias_r = bias_r + K(2) * y;
angle = roll;

I = [1 0; 0 1];
P_temp = (I - K*H)*P_temp;
P = P_temp;

return 


end
